simulink model "Battery_Model"  (R2019b)
settings: configuration reference "BMS_Sw_CodeGenConfig" (kept outside this file)
undefined symbols (not defined in the file): Battery, TempInit, ts
libraries: fl_lib x2765, nesl_utility x1565, ee_lib x384, simulink x384, BatteryPack_lib x3
(part 22 of 33)

== system Battery_Model/Battery_Pack/Battery_Pack_7Modules/Cell_3p05/CellMonitoringUnit_1 ==
  BalCmd : Inport
  D{1..4,7..9,13..16} (11 alike) : fl_lib/Electrical/Electrical Elements/Diode  Vf=0.6 V  Ron=0.3 Ohm  Goff=1e-8 1/Ohm  i_specify=off  i_priority=High  i=0 A  i_nominal_specify=off  i_nominal_unit=A  i_nominal_value=1  v_specify=off  v_priority=None  v=0 V  v_nominal_specify=off  v_nominal_unit=V  v_nominal_value=1
      settings: LogSimulationData=on
  D{5..6,10..12} (5 alike) : fl_lib/Electrical/Electrical Elements/Diode  Vf=0.6 V  Ron=0.3 Ohm  Goff=1e-8 1/Ohm  i_specify=off  i_priority=None  i=0 A  i_nominal_specify=off  i_nominal_unit=A  i_nominal_value=1  v_specify=off  v_priority=None  v=0 V  v_nominal_specify=off  v_nominal_unit=V  v_nominal_value=1
      settings: LogSimulationData=on
  Data Type Conversion{,1..15} (16 alike) : DataTypeConversion  OutDataTypeStr=single
  PS-Simulink Converter{1..12,14..17} (16 alike) : nesl_utility/PS-Simulink Converter  PhysicalDomain=network_engine_domain  SubClassName=ps_output  LeftPortType=input  RightPortType=output  PseudoPeriodic=off  Frequencies=[]  Unit=V  AffineConversion=off
  R{1..16} (16 alike) : fl_lib/Electrical/Electrical Elements/Resistor  R=Battery.R_bleed Ohm  i_specify=off  i_priority=None  i=0 A  i_nominal_specify=off  i_nominal_unit=A  i_nominal_value=1  v_specify=off  v_priority=None  v=0 V  v_nominal_specify=off  v_nominal_unit=V  v_nominal_value=1
      R1 settings: LogSimulationData=on
  Selector : Selector  IndexOptions=Index vector (dialog)  Indices=1  OutputSizes=1
  Selector1 : Selector  IndexOptions=Index vector (dialog)  Indices=2  OutputSizes=1
  Selector10 : Selector  IndexOptions=Index vector (dialog)  Indices=6  OutputSizes=1
  Selector{3,8,11,15} (4 alike) : Selector  IndexOptions=Index vector (dialog)  Indices=4  OutputSizes=1
  Selector12 : Selector  IndexOptions=Index vector (dialog)  Indices=6  OutputSizes=1
  Selector13 : Selector  IndexOptions=Index vector (dialog)  Indices=2  OutputSizes=1
  Selector14 : Selector  IndexOptions=Index vector (dialog)  Indices=3  OutputSizes=1
  Selector2 : Selector  IndexOptions=Index vector (dialog)  Indices=3  OutputSizes=1
  Selector4 : Selector  IndexOptions=Index vector (dialog)  Indices=5  OutputSizes=1
  Selector5 : Selector  IndexOptions=Index vector (dialog)  Indices=6  OutputSizes=1
  Selector6 : Selector  IndexOptions=Index vector (dialog)  Indices=2  OutputSizes=1
  Selector7 : Selector  IndexOptions=Index vector (dialog)  Indices=3  OutputSizes=1
  Selector9 : Selector  IndexOptions=Index vector (dialog)  Indices=5  OutputSizes=1
  Simulink-PS Converter{1..12,14..17} (16 alike) : nesl_utility/Simulink-PS Converter  PhysicalDomain=network_engine_domain  SubClassName=ps_input  LeftPortType=input  RightPortType=output  PseudoPeriodic=off  Frequencies=[]  NoiseDistribution=none  NoiseParameters=[]  Unit=1  AffineConversion=off  FilteringAndDerivatives=zero  SimscapeFilterOrder=1  InputFilterTimeConstant=0.001  UdotUserProvided=1
  Switch{,1..15} (16 alike) : fl_lib/Electrical/Electrical Elements/Switch  R_closed=0.01 Ohm  G_open=1e-8 1/Ohm  Threshold=0  i_specify=off  i_priority=None  i=0 A  i_nominal_specify=off  i_nominal_unit=A  i_nominal_value=1  v_specify=off  v_priority=None  v=0 V  v_nominal_specify=off  v_nominal_unit=V  v_nominal_value=1
      settings: SourceProductName=Simscape
  Vector Concatenate : Concatenate  NumInputs=16
  Voltage Sensor{1..12,14..17} (16 alike) : fl_lib/Electrical/Electrical Sensors/Voltage Sensor
  Conn1 : PMIOPort  Side=Left
  Conn2 : PMIOPort  Port=2  Side=Left
  Conn3 : PMIOPort  Port=3  Side=Left
  Conn4 : PMIOPort  Port=4  Side=Left
  Conn5 : PMIOPort  Port=5  Side=Left
  Conn6 : PMIOPort  Port=6  Side=Left
  Conn7 : PMIOPort  Port=7  Side=Left
  Conn8 : PMIOPort  Port=8  Side=Left
  Conn9 : PMIOPort  Port=9  Side=Left
  Conn10 : PMIOPort  Port=10  Side=Left
  Conn11 : PMIOPort  Port=11  Side=Left
  Conn12 : PMIOPort  Port=12  Side=Left
  Conn13 : PMIOPort  Port=13  Side=Left
  Conn14 : PMIOPort  Port=14  Side=Left
  Conn15 : PMIOPort  Port=15  Side=Left
  Conn16 : PMIOPort  Port=16  Side=Left
  Conn17 : PMIOPort  Port=17  Side=Left
  CellVoltages : Outport  VectorParamsAs1DForOutWhenUnconnected=off
  wires:
  Data Type Conversion10/1 -> Vector Concatenate/11  "Cell11_Volt"
  Data Type Conversion6/1 -> Vector Concatenate/7  "Cell7_Volt"
  Data Type Conversion5/1 -> Vector Concatenate/6  "Cell6_Volt"
  PS-Simulink Converter5/1 -> Data Type Conversion4/1  "Cell5_Volt"
  PS-Simulink Converter3/1 -> Data Type Conversion3/1  "Cell4_Volt"
  Selector/1 -> Simulink-PS Converter3/1
  PS-Simulink Converter1/1 -> Data Type Conversion2/1  "Cell3_Volt"
  Selector3/1 -> Simulink-PS Converter2/1
  PS-Simulink Converter2/1 -> Data Type Conversion/1  "Cell1_Volt"
  Selector1/1 -> Simulink-PS Converter1/1
  Selector4/1 -> Simulink-PS Converter5/1
  Vector Concatenate/1 -> CellVoltages/1
  Data Type Conversion14/1 -> Vector Concatenate/14  "Cell14_Volt"
  Selector11/1 -> Simulink-PS Converter12/1
  PS-Simulink Converter4/1 -> Data Type Conversion1/1  "Cell2_Volt"
  PS-Simulink Converter6/1 -> Data Type Conversion5/1  "Cell6_Volt"
  Data Type Conversion9/1 -> Vector Concatenate/10  "Cell10_Volt"
  Data Type Conversion1/1 -> Vector Concatenate/2  "Cell2_Volt"
  Selector13/1 -> Simulink-PS Converter15/1
  PS-Simulink Converter16/1 -> Data Type Conversion15/1  "Cell15_Volt"
  Data Type Conversion13/1 -> Vector Concatenate/13  "Cell13_Volt"
  PS-Simulink Converter17/1 -> Data Type Conversion13/1  "Cell13_Volt"
  Selector14/1 -> Simulink-PS Converter17/1
  Selector15/1 -> Simulink-PS Converter16/1
  PS-Simulink Converter14/1 -> Data Type Conversion12/1  "Cell12_Volt"
  Selector12/1 -> Simulink-PS Converter14/1
  Selector7/1 -> Simulink-PS Converter9/1
  PS-Simulink Converter7/1 -> Data Type Conversion7/1  "Cell8_Volt"
  Data Type Conversion7/1 -> Vector Concatenate/8  "Cell8_Volt"
  Data Type Conversion2/1 -> Vector Concatenate/3  "Cell3_Volt"
  PS-Simulink Converter11/1 -> Data Type Conversion10/1  "Cell11_Volt"
  PS-Simulink Converter9/1 -> Data Type Conversion6/1  "Cell7_Volt"
  Data Type Conversion4/1 -> Vector Concatenate/5  "Cell5_Volt"
  PS-Simulink Converter15/1 -> Data Type Conversion14/1  "Cell14_Volt"
  Selector10/1 -> Simulink-PS Converter11/1
  Data Type Conversion11/1 -> Vector Concatenate/16  "Cell16_Volt"
  Data Type Conversion15/1 -> Vector Concatenate/15  "Cell15_Volt"
  Selector8/1 -> Simulink-PS Converter8/1
  Data Type Conversion/1 -> Vector Concatenate/1  "Cell1_Volt"
  Selector2/1 -> Simulink-PS Converter4/1
  Data Type Conversion8/1 -> Vector Concatenate/9  "Cell9_Volt"
  PS-Simulink Converter12/1 -> Data Type Conversion11/1  "Cell16_Volt"
  Selector6/1 -> Simulink-PS Converter7/1
  Data Type Conversion12/1 -> Vector Concatenate/12  "Cell12_Volt"
  Data Type Conversion3/1 -> Vector Concatenate/4  "Cell4_Volt"
  Selector9/1 -> Simulink-PS Converter10/1
  PS-Simulink Converter10/1 -> Data Type Conversion9/1  "Cell10_Volt"
  Selector5/1 -> Simulink-PS Converter6/1
  PS-Simulink Converter8/1 -> Data Type Conversion8/1  "Cell9_Volt"
  BalCmd/1 -> Selector2/1, Selector3/1, Selector4/1, Selector5/1, Selector6/1, Selector7/1, Selector8/1, Selector9/1, Selector10/1, Selector12/1, Selector13/1, Selector14/1, Selector15/1, Selector11/1, Selector1/1, Selector/1
  connections:
  Switch11/LConn1 -- D16/RConn1
  R16/RConn1 -- D16/LConn1
  Switch10/LConn1 -- D11/RConn1
  Simulink-PS Converter11/RConn1 -- Switch10/RConn1
  Voltage Sensor6/RConn1 -- PS-Simulink Converter6/LConn1
  R10/RConn1 -- D10/LConn1
  Voltage Sensor5/RConn1 -- PS-Simulink Converter5/LConn1
  R6/RConn1 -- D6/LConn1
  Switch/LConn1 -- D1/RConn1
  Voltage Sensor3/RConn1 -- PS-Simulink Converter1/LConn1
  R5/RConn1 -- D5/LConn1
  R1/RConn1 -- D1/LConn1
  Voltage Sensor2/RConn1 -- PS-Simulink Converter4/LConn1
  Switch4/LConn1 -- D5/RConn1
  Simulink-PS Converter3/RConn1 -- Switch/RConn1
  Switch2/LConn1 -- D3/RConn1
  Simulink-PS Converter5/RConn1 -- Switch4/RConn1
  R2/RConn1 -- D2/LConn1
  Switch1/LConn1 -- D2/RConn1
  R4/RConn1 -- D4/LConn1
  PS-Simulink Converter2/LConn1 -- Voltage Sensor1/RConn1
  Simulink-PS Converter1/RConn1 -- Switch1/RConn1
  Simulink-PS Converter12/RConn1 -- Switch11/RConn1
  Conn3/RConn1 -- Switch1/RConn2 -- R3/LConn1 -- Voltage Sensor2/RConn2 -- Voltage Sensor3/LConn1
  Conn1/RConn1 -- Voltage Sensor1/LConn1 -- R1/LConn1
  Voltage Sensor8/RConn1 -- PS-Simulink Converter7/LConn1
  Conn9/RConn1 -- Voltage Sensor8/RConn2 -- Voltage Sensor9/LConn1 -- R9/LConn1 -- Switch7/RConn2
  Switch5/LConn1 -- D6/RConn1
  Simulink-PS Converter15/RConn1 -- Switch13/RConn1
  R15/RConn1 -- D15/LConn1
  Conn17/RConn1 -- Voltage Sensor12/RConn2 -- Switch11/RConn2
  Voltage Sensor15/RConn1 -- PS-Simulink Converter17/LConn1
  Switch14/LConn1 -- D14/RConn1
  R13/RConn1 -- D13/LConn1
  Simulink-PS Converter2/RConn1 -- Switch3/RConn1
  Switch12/LConn1 -- D12/RConn1
  Conn15/RConn1 -- Voltage Sensor16/RConn2 -- Voltage Sensor17/LConn1 -- R15/LConn1 -- Switch14/RConn2
  Simulink-PS Converter17/RConn1 -- Switch14/RConn1
  R14/RConn1 -- D14/LConn1
  Simulink-PS Converter14/RConn1 -- Switch12/RConn1
  Voltage Sensor11/RConn1 -- PS-Simulink Converter11/LConn1
  R12/RConn1 -- D12/LConn1
  Conn4/RConn1 -- Voltage Sensor3/RConn2 -- Voltage Sensor4/LConn1 -- R4/LConn1 -- Switch2/RConn2
  Conn7/RConn1 -- Switch5/RConn2 -- R7/LConn1 -- Voltage Sensor6/RConn2 -- Voltage Sensor7/LConn1
  Conn10/RConn1 -- Switch8/RConn2 -- R10/LConn1 -- Voltage Sensor10/LConn1 -- Voltage Sensor9/RConn2
  Switch15/LConn1 -- D15/RConn1
  Conn2/RConn1 -- Voltage Sensor1/RConn2 -- Voltage Sensor2/LConn1 -- R2/LConn1 -- Switch/RConn2
  Conn8/RConn1 -- Voltage Sensor8/LConn1 -- Voltage Sensor7/RConn2 -- R8/LConn1 -- Switch6/RConn2
  Switch3/LConn1 -- D4/RConn1
  Voltage Sensor17/RConn1 -- PS-Simulink Converter16/LConn1
  Conn6/RConn1 -- R6/LConn1 -- Voltage Sensor5/RConn2 -- Voltage Sensor6/LConn1 -- Switch4/RConn2
  Switch6/LConn1 -- D7/RConn1
  R3/RConn1 -- D3/LConn1
  Simulink-PS Converter8/RConn1 -- Switch8/RConn1
  Switch8/LConn1 -- D9/RConn1
  R7/RConn1 -- D7/LConn1
  Simulink-PS Converter9/RConn1 -- Switch7/RConn1
  Simulink-PS Converter6/RConn1 -- Switch5/RConn1
  Voltage Sensor16/RConn1 -- PS-Simulink Converter15/LConn1
  R9/RConn1 -- D9/LConn1
  R8/RConn1 -- D8/LConn1
  Switch9/LConn1 -- D10/RConn1
  Voltage Sensor9/RConn1 -- PS-Simulink Converter8/LConn1
  Voltage Sensor7/RConn1 -- PS-Simulink Converter9/LConn1
  Voltage Sensor14/RConn1 -- PS-Simulink Converter14/LConn1
  R11/RConn1 -- D11/LConn1
  Simulink-PS Converter7/RConn1 -- Switch6/RConn1
  Simulink-PS Converter4/RConn1 -- Switch2/RConn1
  Conn12/RConn1 -- Switch10/RConn2 -- R12/LConn1 -- Voltage Sensor11/RConn2 -- Voltage Sensor14/LConn1
  Voltage Sensor12/RConn1 -- PS-Simulink Converter12/LConn1
  Conn14/RConn1 -- Voltage Sensor15/RConn2 -- Voltage Sensor16/LConn1 -- R14/LConn1 -- Switch13/RConn2
  Voltage Sensor4/RConn1 -- PS-Simulink Converter3/LConn1
  Switch13/LConn1 -- D13/RConn1
  Simulink-PS Converter10/RConn1 -- Switch9/RConn1
  Switch7/LConn1 -- D8/RConn1
  Conn11/RConn1 -- Voltage Sensor10/RConn2 -- Voltage Sensor11/LConn1 -- R11/LConn1 -- Switch9/RConn2
  Conn13/RConn1 -- R13/LConn1 -- Voltage Sensor14/RConn2 -- Voltage Sensor15/LConn1 -- Switch12/RConn2
  Conn5/RConn1 -- Switch3/RConn2 -- Voltage Sensor4/RConn2 -- Voltage Sensor5/LConn1 -- R5/LConn1
  Conn16/RConn1 -- R16/LConn1 -- Voltage Sensor17/RConn2 -- Voltage Sensor12/LConn1 -- Switch15/RConn2
  Simulink-PS Converter16/RConn1 -- Switch15/RConn1
  Voltage Sensor10/RConn1 -- PS-Simulink Converter10/LConn1

== system Battery_Model/Battery_Pack/Battery_Pack_7Modules/Cell_3p05/CellMonitoringUnit_2 ==
  BalCmd : Inport
  D{1..4,7..9,13..16} (11 alike) : fl_lib/Electrical/Electrical Elements/Diode  Vf=0.6 V  Ron=0.3 Ohm  Goff=1e-8 1/Ohm  i_specify=off  i_priority=High  i=0 A  i_nominal_specify=off  i_nominal_unit=A  i_nominal_value=1  v_specify=off  v_priority=None  v=0 V  v_nominal_specify=off  v_nominal_unit=V  v_nominal_value=1
      settings: LogSimulationData=on
  D{5..6,10..12} (5 alike) : fl_lib/Electrical/Electrical Elements/Diode  Vf=0.6 V  Ron=0.3 Ohm  Goff=1e-8 1/Ohm  i_specify=off  i_priority=None  i=0 A  i_nominal_specify=off  i_nominal_unit=A  i_nominal_value=1  v_specify=off  v_priority=None  v=0 V  v_nominal_specify=off  v_nominal_unit=V  v_nominal_value=1
      settings: LogSimulationData=on
  Data Type Conversion{,1..15} (16 alike) : DataTypeConversion  OutDataTypeStr=single
  PS-Simulink Converter{1..12,14..17} (16 alike) : nesl_utility/PS-Simulink Converter  PhysicalDomain=network_engine_domain  SubClassName=ps_output  LeftPortType=input  RightPortType=output  PseudoPeriodic=off  Frequencies=[]  Unit=V  AffineConversion=off
  R{1..16} (16 alike) : fl_lib/Electrical/Electrical Elements/Resistor  R=Battery.R_bleed Ohm  i_specify=off  i_priority=None  i=0 A  i_nominal_specify=off  i_nominal_unit=A  i_nominal_value=1  v_specify=off  v_priority=None  v=0 V  v_nominal_specify=off  v_nominal_unit=V  v_nominal_value=1
      R1 settings: LogSimulationData=on
  Selector : Selector  IndexOptions=Index vector (dialog)  Indices=1  OutputSizes=1
  Selector1 : Selector  IndexOptions=Index vector (dialog)  Indices=2  OutputSizes=1
  Selector10 : Selector  IndexOptions=Index vector (dialog)  Indices=6  OutputSizes=1
  Selector{3,8,11,15} (4 alike) : Selector  IndexOptions=Index vector (dialog)  Indices=4  OutputSizes=1
  Selector12 : Selector  IndexOptions=Index vector (dialog)  Indices=6  OutputSizes=1
  Selector13 : Selector  IndexOptions=Index vector (dialog)  Indices=2  OutputSizes=1
  Selector14 : Selector  IndexOptions=Index vector (dialog)  Indices=3  OutputSizes=1
  Selector2 : Selector  IndexOptions=Index vector (dialog)  Indices=3  OutputSizes=1
  Selector4 : Selector  IndexOptions=Index vector (dialog)  Indices=5  OutputSizes=1
  Selector5 : Selector  IndexOptions=Index vector (dialog)  Indices=6  OutputSizes=1
  Selector6 : Selector  IndexOptions=Index vector (dialog)  Indices=2  OutputSizes=1
  Selector7 : Selector  IndexOptions=Index vector (dialog)  Indices=3  OutputSizes=1
  Selector9 : Selector  IndexOptions=Index vector (dialog)  Indices=5  OutputSizes=1
  Simulink-PS Converter{1..12,14..17} (16 alike) : nesl_utility/Simulink-PS Converter  PhysicalDomain=network_engine_domain  SubClassName=ps_input  LeftPortType=input  RightPortType=output  PseudoPeriodic=off  Frequencies=[]  NoiseDistribution=none  NoiseParameters=[]  Unit=1  AffineConversion=off  FilteringAndDerivatives=zero  SimscapeFilterOrder=1  InputFilterTimeConstant=0.001  UdotUserProvided=1
  Switch{,1..15} (16 alike) : fl_lib/Electrical/Electrical Elements/Switch  R_closed=0.01 Ohm  G_open=1e-8 1/Ohm  Threshold=0  i_specify=off  i_priority=None  i=0 A  i_nominal_specify=off  i_nominal_unit=A  i_nominal_value=1  v_specify=off  v_priority=None  v=0 V  v_nominal_specify=off  v_nominal_unit=V  v_nominal_value=1
      settings: SourceProductName=Simscape
  Vector Concatenate : Concatenate  NumInputs=16
  Voltage Sensor{1..12,14..17} (16 alike) : fl_lib/Electrical/Electrical Sensors/Voltage Sensor
  Conn1 : PMIOPort  Side=Left
  Conn2 : PMIOPort  Port=2  Side=Left
  Conn3 : PMIOPort  Port=3  Side=Left
  Conn4 : PMIOPort  Port=4  Side=Left
  Conn5 : PMIOPort  Port=5  Side=Left
  Conn6 : PMIOPort  Port=6  Side=Left
  Conn7 : PMIOPort  Port=7  Side=Left
  Conn8 : PMIOPort  Port=8  Side=Left
  Conn9 : PMIOPort  Port=9  Side=Left
  Conn10 : PMIOPort  Port=10  Side=Left
  Conn11 : PMIOPort  Port=11  Side=Left
  Conn12 : PMIOPort  Port=12  Side=Left
  Conn13 : PMIOPort  Port=13  Side=Left
  Conn14 : PMIOPort  Port=14  Side=Left
  Conn15 : PMIOPort  Port=15  Side=Left
  Conn16 : PMIOPort  Port=16  Side=Left
  Conn17 : PMIOPort  Port=17  Side=Left
  CellVoltages : Outport  VectorParamsAs1DForOutWhenUnconnected=off
  wires:
  Data Type Conversion10/1 -> Vector Concatenate/11  "Cell11_Volt"
  Data Type Conversion6/1 -> Vector Concatenate/7  "Cell7_Volt"
  Data Type Conversion5/1 -> Vector Concatenate/6  "Cell6_Volt"
  PS-Simulink Converter5/1 -> Data Type Conversion4/1  "Cell5_Volt"
  PS-Simulink Converter3/1 -> Data Type Conversion3/1  "Cell4_Volt"
  Selector/1 -> Simulink-PS Converter3/1
  PS-Simulink Converter1/1 -> Data Type Conversion2/1  "Cell3_Volt"
  Selector3/1 -> Simulink-PS Converter2/1
  PS-Simulink Converter2/1 -> Data Type Conversion/1  "Cell1_Volt"
  Selector1/1 -> Simulink-PS Converter1/1
  Selector4/1 -> Simulink-PS Converter5/1
  Vector Concatenate/1 -> CellVoltages/1
  Data Type Conversion14/1 -> Vector Concatenate/14  "Cell14_Volt"
  Selector11/1 -> Simulink-PS Converter12/1
  PS-Simulink Converter4/1 -> Data Type Conversion1/1  "Cell2_Volt"
  PS-Simulink Converter6/1 -> Data Type Conversion5/1  "Cell6_Volt"
  Data Type Conversion9/1 -> Vector Concatenate/10  "Cell10_Volt"
  Data Type Conversion1/1 -> Vector Concatenate/2  "Cell2_Volt"
  Selector13/1 -> Simulink-PS Converter15/1
  PS-Simulink Converter16/1 -> Data Type Conversion15/1  "Cell15_Volt"
  Data Type Conversion13/1 -> Vector Concatenate/13  "Cell13_Volt"
  PS-Simulink Converter17/1 -> Data Type Conversion13/1  "Cell13_Volt"
  Selector14/1 -> Simulink-PS Converter17/1
  Selector15/1 -> Simulink-PS Converter16/1
  PS-Simulink Converter14/1 -> Data Type Conversion12/1  "Cell12_Volt"
  Selector12/1 -> Simulink-PS Converter14/1
  Selector7/1 -> Simulink-PS Converter9/1
  PS-Simulink Converter7/1 -> Data Type Conversion7/1  "Cell8_Volt"
  Data Type Conversion7/1 -> Vector Concatenate/8  "Cell8_Volt"
  Data Type Conversion2/1 -> Vector Concatenate/3  "Cell3_Volt"
  PS-Simulink Converter11/1 -> Data Type Conversion10/1  "Cell11_Volt"
  PS-Simulink Converter9/1 -> Data Type Conversion6/1  "Cell7_Volt"
  Data Type Conversion4/1 -> Vector Concatenate/5  "Cell5_Volt"
  PS-Simulink Converter15/1 -> Data Type Conversion14/1  "Cell14_Volt"
  Selector10/1 -> Simulink-PS Converter11/1
  Data Type Conversion11/1 -> Vector Concatenate/16  "Cell16_Volt"
  Data Type Conversion15/1 -> Vector Concatenate/15  "Cell15_Volt"
  Selector8/1 -> Simulink-PS Converter8/1
  Data Type Conversion/1 -> Vector Concatenate/1  "Cell1_Volt"
  Selector2/1 -> Simulink-PS Converter4/1
  Data Type Conversion8/1 -> Vector Concatenate/9  "Cell9_Volt"
  PS-Simulink Converter12/1 -> Data Type Conversion11/1  "Cell16_Volt"
  Selector6/1 -> Simulink-PS Converter7/1
  Data Type Conversion12/1 -> Vector Concatenate/12  "Cell12_Volt"
  Data Type Conversion3/1 -> Vector Concatenate/4  "Cell4_Volt"
  Selector9/1 -> Simulink-PS Converter10/1
  PS-Simulink Converter10/1 -> Data Type Conversion9/1  "Cell10_Volt"
  Selector5/1 -> Simulink-PS Converter6/1
  PS-Simulink Converter8/1 -> Data Type Conversion8/1  "Cell9_Volt"
  BalCmd/1 -> Selector2/1, Selector3/1, Selector4/1, Selector5/1, Selector6/1, Selector7/1, Selector8/1, Selector9/1, Selector10/1, Selector12/1, Selector13/1, Selector14/1, Selector15/1, Selector11/1, Selector1/1, Selector/1
  connections:
  Switch11/LConn1 -- D16/RConn1
  R16/RConn1 -- D16/LConn1
  Switch10/LConn1 -- D11/RConn1
  Simulink-PS Converter11/RConn1 -- Switch10/RConn1
  Voltage Sensor6/RConn1 -- PS-Simulink Converter6/LConn1
  R10/RConn1 -- D10/LConn1
  Voltage Sensor5/RConn1 -- PS-Simulink Converter5/LConn1
  R6/RConn1 -- D6/LConn1
  Switch/LConn1 -- D1/RConn1
  Voltage Sensor3/RConn1 -- PS-Simulink Converter1/LConn1
  R5/RConn1 -- D5/LConn1
  R1/RConn1 -- D1/LConn1
  Voltage Sensor2/RConn1 -- PS-Simulink Converter4/LConn1
  Switch4/LConn1 -- D5/RConn1
  Simulink-PS Converter3/RConn1 -- Switch/RConn1
  Switch2/LConn1 -- D3/RConn1
  Simulink-PS Converter5/RConn1 -- Switch4/RConn1
  R2/RConn1 -- D2/LConn1
  Switch1/LConn1 -- D2/RConn1
  R4/RConn1 -- D4/LConn1
  PS-Simulink Converter2/LConn1 -- Voltage Sensor1/RConn1
  Simulink-PS Converter1/RConn1 -- Switch1/RConn1
  Simulink-PS Converter12/RConn1 -- Switch11/RConn1
  Conn3/RConn1 -- Switch1/RConn2 -- R3/LConn1 -- Voltage Sensor2/RConn2 -- Voltage Sensor3/LConn1
  Conn1/RConn1 -- Voltage Sensor1/LConn1 -- R1/LConn1
  Voltage Sensor8/RConn1 -- PS-Simulink Converter7/LConn1
  Conn9/RConn1 -- Voltage Sensor8/RConn2 -- Voltage Sensor9/LConn1 -- R9/LConn1 -- Switch7/RConn2
  Switch5/LConn1 -- D6/RConn1
  Simulink-PS Converter15/RConn1 -- Switch13/RConn1
  R15/RConn1 -- D15/LConn1
  Conn17/RConn1 -- Voltage Sensor12/RConn2 -- Switch11/RConn2
  Voltage Sensor15/RConn1 -- PS-Simulink Converter17/LConn1
  Switch14/LConn1 -- D14/RConn1
  R13/RConn1 -- D13/LConn1
  Simulink-PS Converter2/RConn1 -- Switch3/RConn1
  Switch12/LConn1 -- D12/RConn1
  Conn15/RConn1 -- Voltage Sensor16/RConn2 -- Voltage Sensor17/LConn1 -- R15/LConn1 -- Switch14/RConn2
  Simulink-PS Converter17/RConn1 -- Switch14/RConn1
  R14/RConn1 -- D14/LConn1
  Simulink-PS Converter14/RConn1 -- Switch12/RConn1
  Voltage Sensor11/RConn1 -- PS-Simulink Converter11/LConn1
  R12/RConn1 -- D12/LConn1
  Conn4/RConn1 -- Voltage Sensor3/RConn2 -- Voltage Sensor4/LConn1 -- R4/LConn1 -- Switch2/RConn2
  Conn7/RConn1 -- Switch5/RConn2 -- R7/LConn1 -- Voltage Sensor6/RConn2 -- Voltage Sensor7/LConn1
  Conn10/RConn1 -- Switch8/RConn2 -- R10/LConn1 -- Voltage Sensor10/LConn1 -- Voltage Sensor9/RConn2
  Switch15/LConn1 -- D15/RConn1
  Conn2/RConn1 -- Voltage Sensor1/RConn2 -- Voltage Sensor2/LConn1 -- R2/LConn1 -- Switch/RConn2
  Conn8/RConn1 -- Voltage Sensor8/LConn1 -- Voltage Sensor7/RConn2 -- R8/LConn1 -- Switch6/RConn2
  Switch3/LConn1 -- D4/RConn1
  Voltage Sensor17/RConn1 -- PS-Simulink Converter16/LConn1
  Conn6/RConn1 -- R6/LConn1 -- Voltage Sensor5/RConn2 -- Voltage Sensor6/LConn1 -- Switch4/RConn2
  Switch6/LConn1 -- D7/RConn1
  R3/RConn1 -- D3/LConn1
  Simulink-PS Converter8/RConn1 -- Switch8/RConn1
  Switch8/LConn1 -- D9/RConn1
  R7/RConn1 -- D7/LConn1
  Simulink-PS Converter9/RConn1 -- Switch7/RConn1
  Simulink-PS Converter6/RConn1 -- Switch5/RConn1
  Voltage Sensor16/RConn1 -- PS-Simulink Converter15/LConn1
  R9/RConn1 -- D9/LConn1
  R8/RConn1 -- D8/LConn1
  Switch9/LConn1 -- D10/RConn1
  Voltage Sensor9/RConn1 -- PS-Simulink Converter8/LConn1
  Voltage Sensor7/RConn1 -- PS-Simulink Converter9/LConn1
  Voltage Sensor14/RConn1 -- PS-Simulink Converter14/LConn1
  R11/RConn1 -- D11/LConn1
  Simulink-PS Converter7/RConn1 -- Switch6/RConn1
  Simulink-PS Converter4/RConn1 -- Switch2/RConn1
  Conn12/RConn1 -- Switch10/RConn2 -- R12/LConn1 -- Voltage Sensor11/RConn2 -- Voltage Sensor14/LConn1
  Voltage Sensor12/RConn1 -- PS-Simulink Converter12/LConn1
  Conn14/RConn1 -- Voltage Sensor15/RConn2 -- Voltage Sensor16/LConn1 -- R14/LConn1 -- Switch13/RConn2
  Voltage Sensor4/RConn1 -- PS-Simulink Converter3/LConn1
  Switch13/LConn1 -- D13/RConn1
  Simulink-PS Converter10/RConn1 -- Switch9/RConn1
  Switch7/LConn1 -- D8/RConn1
  Conn11/RConn1 -- Voltage Sensor10/RConn2 -- Voltage Sensor11/LConn1 -- R11/LConn1 -- Switch9/RConn2
  Conn13/RConn1 -- R13/LConn1 -- Voltage Sensor14/RConn2 -- Voltage Sensor15/LConn1 -- Switch12/RConn2
  Conn5/RConn1 -- Switch3/RConn2 -- Voltage Sensor4/RConn2 -- Voltage Sensor5/LConn1 -- R5/LConn1
  Conn16/RConn1 -- R16/LConn1 -- Voltage Sensor17/RConn2 -- Voltage Sensor12/LConn1 -- Switch15/RConn2
  Simulink-PS Converter16/RConn1 -- Switch15/RConn1
  Voltage Sensor10/RConn1 -- PS-Simulink Converter10/LConn1

== system Battery_Model/Battery_Pack/Battery_Pack_7Modules/Cell_3p05/CellMonitoringUnit_3 ==
  BalCmd : Inport
  D{1..4,7..9,13..16} (11 alike) : fl_lib/Electrical/Electrical Elements/Diode  Vf=0.6 V  Ron=0.3 Ohm  Goff=1e-8 1/Ohm  i_specify=off  i_priority=High  i=0 A  i_nominal_specify=off  i_nominal_unit=A  i_nominal_value=1  v_specify=off  v_priority=None  v=0 V  v_nominal_specify=off  v_nominal_unit=V  v_nominal_value=1
      settings: LogSimulationData=on
  D{5..6,10..12} (5 alike) : fl_lib/Electrical/Electrical Elements/Diode  Vf=0.6 V  Ron=0.3 Ohm  Goff=1e-8 1/Ohm  i_specify=off  i_priority=None  i=0 A  i_nominal_specify=off  i_nominal_unit=A  i_nominal_value=1  v_specify=off  v_priority=None  v=0 V  v_nominal_specify=off  v_nominal_unit=V  v_nominal_value=1
      settings: LogSimulationData=on
  Data Type Conversion{,1..15} (16 alike) : DataTypeConversion  OutDataTypeStr=single
  PS-Simulink Converter{1..12,14..17} (16 alike) : nesl_utility/PS-Simulink Converter  PhysicalDomain=network_engine_domain  SubClassName=ps_output  LeftPortType=input  RightPortType=output  PseudoPeriodic=off  Frequencies=[]  Unit=V  AffineConversion=off
  R{1..16} (16 alike) : fl_lib/Electrical/Electrical Elements/Resistor  R=Battery.R_bleed Ohm  i_specify=off  i_priority=None  i=0 A  i_nominal_specify=off  i_nominal_unit=A  i_nominal_value=1  v_specify=off  v_priority=None  v=0 V  v_nominal_specify=off  v_nominal_unit=V  v_nominal_value=1
      R1 settings: LogSimulationData=on
  Selector : Selector  IndexOptions=Index vector (dialog)  Indices=1  OutputSizes=1
  Selector1 : Selector  IndexOptions=Index vector (dialog)  Indices=2  OutputSizes=1
  Selector10 : Selector  IndexOptions=Index vector (dialog)  Indices=6  OutputSizes=1
  Selector{3,8,11,15} (4 alike) : Selector  IndexOptions=Index vector (dialog)  Indices=4  OutputSizes=1
  Selector12 : Selector  IndexOptions=Index vector (dialog)  Indices=6  OutputSizes=1
  Selector13 : Selector  IndexOptions=Index vector (dialog)  Indices=2  OutputSizes=1
  Selector14 : Selector  IndexOptions=Index vector (dialog)  Indices=3  OutputSizes=1
  Selector2 : Selector  IndexOptions=Index vector (dialog)  Indices=3  OutputSizes=1
  Selector4 : Selector  IndexOptions=Index vector (dialog)  Indices=5  OutputSizes=1
  Selector5 : Selector  IndexOptions=Index vector (dialog)  Indices=6  OutputSizes=1
  Selector6 : Selector  IndexOptions=Index vector (dialog)  Indices=2  OutputSizes=1
  Selector7 : Selector  IndexOptions=Index vector (dialog)  Indices=3  OutputSizes=1
  Selector9 : Selector  IndexOptions=Index vector (dialog)  Indices=5  OutputSizes=1
  Simulink-PS Converter{1..12,14..17} (16 alike) : nesl_utility/Simulink-PS Converter  PhysicalDomain=network_engine_domain  SubClassName=ps_input  LeftPortType=input  RightPortType=output  PseudoPeriodic=off  Frequencies=[]  NoiseDistribution=none  NoiseParameters=[]  Unit=1  AffineConversion=off  FilteringAndDerivatives=zero  SimscapeFilterOrder=1  InputFilterTimeConstant=0.001  UdotUserProvided=1
  Switch{,1..15} (16 alike) : fl_lib/Electrical/Electrical Elements/Switch  R_closed=0.01 Ohm  G_open=1e-8 1/Ohm  Threshold=0  i_specify=off  i_priority=None  i=0 A  i_nominal_specify=off  i_nominal_unit=A  i_nominal_value=1  v_specify=off  v_priority=None  v=0 V  v_nominal_specify=off  v_nominal_unit=V  v_nominal_value=1
      settings: SourceProductName=Simscape
  Vector Concatenate : Concatenate  NumInputs=16
  Voltage Sensor{1..12,14..17} (16 alike) : fl_lib/Electrical/Electrical Sensors/Voltage Sensor
  Conn1 : PMIOPort  Side=Left
  Conn2 : PMIOPort  Port=2  Side=Left
  Conn3 : PMIOPort  Port=3  Side=Left
  Conn4 : PMIOPort  Port=4  Side=Left
  Conn5 : PMIOPort  Port=5  Side=Left
  Conn6 : PMIOPort  Port=6  Side=Left
  Conn7 : PMIOPort  Port=7  Side=Left
  Conn8 : PMIOPort  Port=8  Side=Left
  Conn9 : PMIOPort  Port=9  Side=Left
  Conn10 : PMIOPort  Port=10  Side=Left
  Conn11 : PMIOPort  Port=11  Side=Left
  Conn12 : PMIOPort  Port=12  Side=Left
  Conn13 : PMIOPort  Port=13  Side=Left
  Conn14 : PMIOPort  Port=14  Side=Left
  Conn15 : PMIOPort  Port=15  Side=Left
  Conn16 : PMIOPort  Port=16  Side=Left
  Conn17 : PMIOPort  Port=17  Side=Left
  CellVoltages : Outport  VectorParamsAs1DForOutWhenUnconnected=off
  wires:
  Data Type Conversion10/1 -> Vector Concatenate/11  "Cell11_Volt"
  Data Type Conversion6/1 -> Vector Concatenate/7  "Cell7_Volt"
  Data Type Conversion5/1 -> Vector Concatenate/6  "Cell6_Volt"
  PS-Simulink Converter5/1 -> Data Type Conversion4/1  "Cell5_Volt"
  PS-Simulink Converter3/1 -> Data Type Conversion3/1  "Cell4_Volt"
  Selector/1 -> Simulink-PS Converter3/1
  PS-Simulink Converter1/1 -> Data Type Conversion2/1  "Cell3_Volt"
  Selector3/1 -> Simulink-PS Converter2/1
  PS-Simulink Converter2/1 -> Data Type Conversion/1  "Cell1_Volt"
  Selector1/1 -> Simulink-PS Converter1/1
  Selector4/1 -> Simulink-PS Converter5/1
  Vector Concatenate/1 -> CellVoltages/1
  Data Type Conversion14/1 -> Vector Concatenate/14  "Cell14_Volt"
  Selector11/1 -> Simulink-PS Converter12/1
  PS-Simulink Converter4/1 -> Data Type Conversion1/1  "Cell2_Volt"
  PS-Simulink Converter6/1 -> Data Type Conversion5/1  "Cell6_Volt"
  Data Type Conversion9/1 -> Vector Concatenate/10  "Cell10_Volt"
  Data Type Conversion1/1 -> Vector Concatenate/2  "Cell2_Volt"
  Selector13/1 -> Simulink-PS Converter15/1
  PS-Simulink Converter16/1 -> Data Type Conversion15/1  "Cell15_Volt"
  Data Type Conversion13/1 -> Vector Concatenate/13  "Cell13_Volt"
  PS-Simulink Converter17/1 -> Data Type Conversion13/1  "Cell13_Volt"
  Selector14/1 -> Simulink-PS Converter17/1
  Selector15/1 -> Simulink-PS Converter16/1
  PS-Simulink Converter14/1 -> Data Type Conversion12/1  "Cell12_Volt"
  Selector12/1 -> Simulink-PS Converter14/1
  Selector7/1 -> Simulink-PS Converter9/1
  PS-Simulink Converter7/1 -> Data Type Conversion7/1  "Cell8_Volt"
  Data Type Conversion7/1 -> Vector Concatenate/8  "Cell8_Volt"
  Data Type Conversion2/1 -> Vector Concatenate/3  "Cell3_Volt"
  PS-Simulink Converter11/1 -> Data Type Conversion10/1  "Cell11_Volt"
  PS-Simulink Converter9/1 -> Data Type Conversion6/1  "Cell7_Volt"
  Data Type Conversion4/1 -> Vector Concatenate/5  "Cell5_Volt"
  PS-Simulink Converter15/1 -> Data Type Conversion14/1  "Cell14_Volt"
  Selector10/1 -> Simulink-PS Converter11/1
  Data Type Conversion11/1 -> Vector Concatenate/16  "Cell16_Volt"
  Data Type Conversion15/1 -> Vector Concatenate/15  "Cell15_Volt"
  Selector8/1 -> Simulink-PS Converter8/1
  Data Type Conversion/1 -> Vector Concatenate/1  "Cell1_Volt"
  Selector2/1 -> Simulink-PS Converter4/1
  Data Type Conversion8/1 -> Vector Concatenate/9  "Cell9_Volt"
  PS-Simulink Converter12/1 -> Data Type Conversion11/1  "Cell16_Volt"
  Selector6/1 -> Simulink-PS Converter7/1
  Data Type Conversion12/1 -> Vector Concatenate/12  "Cell12_Volt"
  Data Type Conversion3/1 -> Vector Concatenate/4  "Cell4_Volt"
  Selector9/1 -> Simulink-PS Converter10/1
  PS-Simulink Converter10/1 -> Data Type Conversion9/1  "Cell10_Volt"
  Selector5/1 -> Simulink-PS Converter6/1
  PS-Simulink Converter8/1 -> Data Type Conversion8/1  "Cell9_Volt"
  BalCmd/1 -> Selector2/1, Selector3/1, Selector4/1, Selector5/1, Selector6/1, Selector7/1, Selector8/1, Selector9/1, Selector10/1, Selector12/1, Selector13/1, Selector14/1, Selector15/1, Selector11/1, Selector1/1, Selector/1
  connections:
  Switch11/LConn1 -- D16/RConn1
  R16/RConn1 -- D16/LConn1
  Switch10/LConn1 -- D11/RConn1
  Simulink-PS Converter11/RConn1 -- Switch10/RConn1
  Voltage Sensor6/RConn1 -- PS-Simulink Converter6/LConn1
  R10/RConn1 -- D10/LConn1
  Voltage Sensor5/RConn1 -- PS-Simulink Converter5/LConn1
  R6/RConn1 -- D6/LConn1
  Switch/LConn1 -- D1/RConn1
  Voltage Sensor3/RConn1 -- PS-Simulink Converter1/LConn1
  R5/RConn1 -- D5/LConn1
  R1/RConn1 -- D1/LConn1
  Voltage Sensor2/RConn1 -- PS-Simulink Converter4/LConn1
  Switch4/LConn1 -- D5/RConn1
  Simulink-PS Converter3/RConn1 -- Switch/RConn1
  Switch2/LConn1 -- D3/RConn1
  Simulink-PS Converter5/RConn1 -- Switch4/RConn1
  R2/RConn1 -- D2/LConn1
  Switch1/LConn1 -- D2/RConn1
  R4/RConn1 -- D4/LConn1
  PS-Simulink Converter2/LConn1 -- Voltage Sensor1/RConn1
  Simulink-PS Converter1/RConn1 -- Switch1/RConn1
  Simulink-PS Converter12/RConn1 -- Switch11/RConn1
  Conn3/RConn1 -- Switch1/RConn2 -- R3/LConn1 -- Voltage Sensor2/RConn2 -- Voltage Sensor3/LConn1
  Conn1/RConn1 -- Voltage Sensor1/LConn1 -- R1/LConn1
  Voltage Sensor8/RConn1 -- PS-Simulink Converter7/LConn1
  Conn9/RConn1 -- Voltage Sensor8/RConn2 -- Voltage Sensor9/LConn1 -- R9/LConn1 -- Switch7/RConn2
  Switch5/LConn1 -- D6/RConn1
  Simulink-PS Converter15/RConn1 -- Switch13/RConn1
  R15/RConn1 -- D15/LConn1
  Conn17/RConn1 -- Voltage Sensor12/RConn2 -- Switch11/RConn2
  Voltage Sensor15/RConn1 -- PS-Simulink Converter17/LConn1
  Switch14/LConn1 -- D14/RConn1
  R13/RConn1 -- D13/LConn1
  Simulink-PS Converter2/RConn1 -- Switch3/RConn1
  Switch12/LConn1 -- D12/RConn1
  Conn15/RConn1 -- Voltage Sensor16/RConn2 -- Voltage Sensor17/LConn1 -- R15/LConn1 -- Switch14/RConn2
  Simulink-PS Converter17/RConn1 -- Switch14/RConn1
  R14/RConn1 -- D14/LConn1
  Simulink-PS Converter14/RConn1 -- Switch12/RConn1
  Voltage Sensor11/RConn1 -- PS-Simulink Converter11/LConn1
  R12/RConn1 -- D12/LConn1
  Conn4/RConn1 -- Voltage Sensor3/RConn2 -- Voltage Sensor4/LConn1 -- R4/LConn1 -- Switch2/RConn2
  Conn7/RConn1 -- Switch5/RConn2 -- R7/LConn1 -- Voltage Sensor6/RConn2 -- Voltage Sensor7/LConn1
  Conn10/RConn1 -- Switch8/RConn2 -- R10/LConn1 -- Voltage Sensor10/LConn1 -- Voltage Sensor9/RConn2
  Switch15/LConn1 -- D15/RConn1
  Conn2/RConn1 -- Voltage Sensor1/RConn2 -- Voltage Sensor2/LConn1 -- R2/LConn1 -- Switch/RConn2
  Conn8/RConn1 -- Voltage Sensor8/LConn1 -- Voltage Sensor7/RConn2 -- R8/LConn1 -- Switch6/RConn2
  Switch3/LConn1 -- D4/RConn1
  Voltage Sensor17/RConn1 -- PS-Simulink Converter16/LConn1
  Conn6/RConn1 -- R6/LConn1 -- Voltage Sensor5/RConn2 -- Voltage Sensor6/LConn1 -- Switch4/RConn2
  Switch6/LConn1 -- D7/RConn1
  R3/RConn1 -- D3/LConn1
  Simulink-PS Converter8/RConn1 -- Switch8/RConn1
  Switch8/LConn1 -- D9/RConn1
  R7/RConn1 -- D7/LConn1
  Simulink-PS Converter9/RConn1 -- Switch7/RConn1
  Simulink-PS Converter6/RConn1 -- Switch5/RConn1
  Voltage Sensor16/RConn1 -- PS-Simulink Converter15/LConn1
  R9/RConn1 -- D9/LConn1
  R8/RConn1 -- D8/LConn1
  Switch9/LConn1 -- D10/RConn1
  Voltage Sensor9/RConn1 -- PS-Simulink Converter8/LConn1
  Voltage Sensor7/RConn1 -- PS-Simulink Converter9/LConn1
  Voltage Sensor14/RConn1 -- PS-Simulink Converter14/LConn1
  R11/RConn1 -- D11/LConn1
  Simulink-PS Converter7/RConn1 -- Switch6/RConn1
  Simulink-PS Converter4/RConn1 -- Switch2/RConn1
  Conn12/RConn1 -- Switch10/RConn2 -- R12/LConn1 -- Voltage Sensor11/RConn2 -- Voltage Sensor14/LConn1
  Voltage Sensor12/RConn1 -- PS-Simulink Converter12/LConn1
  Conn14/RConn1 -- Voltage Sensor15/RConn2 -- Voltage Sensor16/LConn1 -- R14/LConn1 -- Switch13/RConn2
  Voltage Sensor4/RConn1 -- PS-Simulink Converter3/LConn1
  Switch13/LConn1 -- D13/RConn1
  Simulink-PS Converter10/RConn1 -- Switch9/RConn1
  Switch7/LConn1 -- D8/RConn1
  Conn11/RConn1 -- Voltage Sensor10/RConn2 -- Voltage Sensor11/LConn1 -- R11/LConn1 -- Switch9/RConn2
  Conn13/RConn1 -- R13/LConn1 -- Voltage Sensor14/RConn2 -- Voltage Sensor15/LConn1 -- Switch12/RConn2
  Conn5/RConn1 -- Switch3/RConn2 -- Voltage Sensor4/RConn2 -- Voltage Sensor5/LConn1 -- R5/LConn1
  Conn16/RConn1 -- R16/LConn1 -- Voltage Sensor17/RConn2 -- Voltage Sensor12/LConn1 -- Switch15/RConn2
  Simulink-PS Converter16/RConn1 -- Switch15/RConn1
  Voltage Sensor10/RConn1 -- PS-Simulink Converter10/LConn1
